simulink model "upsample_ref2"  (Simulink 4.00)
settings: Solver=FixedStepDiscrete  StartTime=0.0  StopTime=5  RelTol=1e-3
PreLoadFcn:
  | load mtlb
PostLoadFcn:
  | set_param(gcs,'SimulationCommand','Update')
libraries: dspsrcs3 x1, dspsigops x1
settings Model: RequirementInfo=9  Creator=ckamachi  LastModifiedBy=ckamachi  LimitDataPoints=off  ExtModeTrigMode=oneshot  ExtModeArmWhenConnect=off  BlockReductionOpt=off

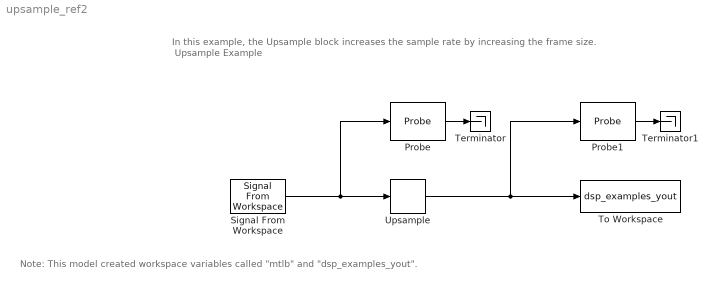
== system upsample_ref2 ==
  note: Upsample Example
  note: In this example, the Upsample block increases the sample rate
      | by increasing the frame size.
  note: Note: This model created workspace variables called "mtlb" and "dsp_examples_yout".
  Probe : Probe  ProbeWidth=off  ProbeSampleTime=on  ProbeComplexSignal=off  ProbeSignalDimensions=off
  Probe1 : Probe  ProbeWidth=off  ProbeSampleTime=on  ProbeComplexSignal=off  ProbeSignalDimensions=off
  Signal From Workspace : dspsrcs3/Signal From Workspace  X=mtlb  Ts=1/16  nsamps=16  OutputAfterFinalValue=Setting To Zero
  Terminator : Terminator
  Terminator1 : Terminator
  To Workspace : ToWorkspace  VariableName=dsp_examples_yout  SampleTime=-1  SaveFormat=Array
  Upsample : dspsigops/Upsample  N=4  phase=0  ic=0  mode=Maintain input frame rate
  wires:
  Upsample/1 -> To Workspace/1, Probe1/1
  Signal From Workspace/1 -> Probe/1, Upsample/1
  Probe/1 -> Terminator/1
  Probe1/1 -> Terminator1/1
